simulink model "simulacion1GDL"  (R2022a)
settings: Solver=VariableStepAuto  StartTime=0.0  StopTime=10.0  RelTol=1e-3
values from neighbouring files (symbols this model uses):
  A = [1;1]    [Pruebas.m]    (also in SDOF_sim.m = [0 1; -k/m -c/m]; Simulacion_1gdl.m = [0 1; -k/m -c/m])
  B = [0; 1]    [SDOF_sim.m]    (also in Simulacion_1gdl.m)
  C = [1 0; 0 1; -k/m -c/m]    [SDOF_sim.m]    (also in Simulacion_1gdl.m)
  D = [0; 0; 0]    [SDOF_sim.m]    (also in Simulacion_1gdl.m)
undefined symbols (not defined in the file or in its folder): x0
settings Model: Creator=LEGION  LastModifiedBy=LEGION

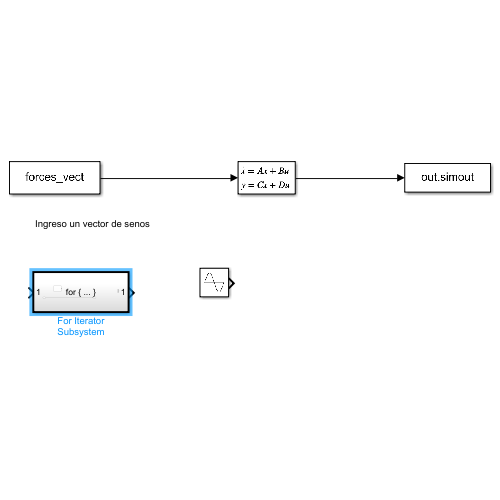
[thumbnail: Simulink's stored preview of the top-level diagram]
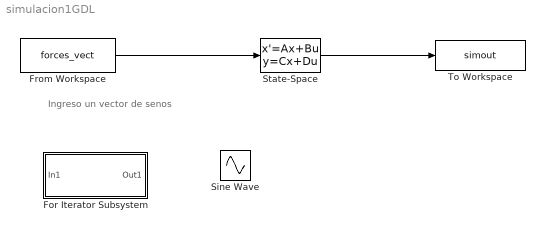
== system simulacion1GDL ==
  note: Ingreso un vector de senos
  For Iterator Subsystem : Subsystem  TreatAsAtomicUnit=on
  From Workspace : FromWorkspace  VariableName=forces_vect  OutputAfterFinalValue=Setting to zero
  Sine Wave : Sin  SampleTime=0
  State-Space : StateSpace  A=A  B=B  C=C  D=D  InitialCondition=x0
  To Workspace : ToWorkspace  VariableName=simout  SaveFormat=Timeseries  SampleTime=-1
  wires:
  From Workspace/1 -> State-Space/1
  State-Space/1 -> To Workspace/1

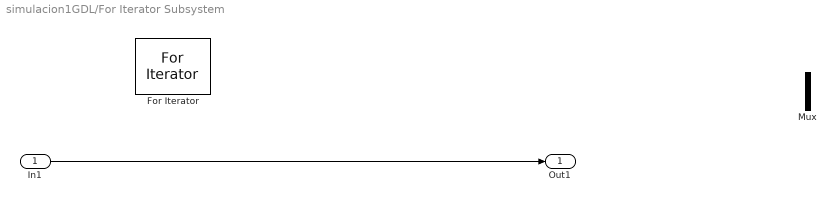
== system simulacion1GDL/For Iterator Subsystem ==
  In1 : Inport
  For Iterator : ForIterator
  Mux : Mux  Inputs=2
  Out1 : Outport
  wires:
  In1/1 -> Out1/1
